simulink model "setPID"  (R2016a)
settings: Solver=FixedStepDiscrete  StartTime=0.0  StopTime=inf  FixedStep=0.005  RelTol=1e-3
PreLoadFcn:
  | if ~exist('Ts', 'var')
  | Ts = 0.001;
  | end
  | if ~exist('Tpwm', 'var')
  | Tpwm = 0.005;
  | end
  | if ~exist('FPGA_Frequency', 'var')
  | FPGA_Frequency = 75000000;
  | end
undefined symbols (not defined in the file or in its folder): IO3xx
libraries: speedgoatlib_fpga x6, slrtlib x3, simulink x1
settings Model: Creator=cedric  LastModifiedBy=kqp5516
settings SolverCC: EnableConcurrentExecution=on
settings DataIOCC: SaveFormat=StructureWithTime
settings OptimizationCC: BlockReduction=off  OptimizeBlockIOStorage=off  BufferReuse=off  GlobalBufferReuse=off  ExpressionFolding=off  LocalBlockOutputs=off
settings DebuggingCC: UnderspecifiedInitializationDetection=Classic  MergeDetectMultiDrivingBlocksExec=none  UnconnectedInputMsg=none  UnconnectedOutputMsg=none  UnconnectedLineMsg=none  SFUnexpectedBacktrackingDiag=error  SFNoUnconditionalDefaultTransitionDiag=error
settings HardwareCC: ProdBitPerPointer=32  ProdLargestAtomicFloat=None  ProdWordSize=32  ProdHWDeviceType=Generic->32-bit x86 compatible
settings ModelReferenceCC: PropagateSignalLabelsOutOfModel=off
settings RTWCC: SystemTargetFile=slrt.tlc  TemplateMakefile=slrt_default_tmf  Description=Simulink Real-Time
settings SimulinkRealTimeCC: RL32LogTETModifier=off  xPCisModelTimeout=off  xPCModelTimeoutSecs=20
settings ConfigComp: CovMetricSettings=dwe  CovHtmlReporting=off  CovSaveCumulativeToWorkspaceVar=off  CovSaveSingleToWorkspaceVar=off  CovExternalEMLEnable=on

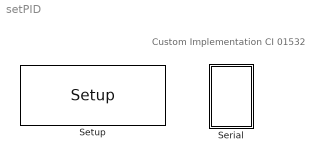
== system setPID ==
  note: Custom Implementation CI 01532
  Serial : Subsystem
  Setup : speedgoatlib_fpga/Setup/Setup  board=IO323  id=1  frontIO=None  rearIO=IO3xx-22  bitstreamFile=speedgoat_IO323_22_CI_01532  ProgSpiFlash=off  ProgBPIFlash=off  pciSlot=-1  PullRPort0=pull-up 3.3V  VioPort0=3.3V  PullRPort1=pull-up 3.3V  VioPort1=3.3V  PullRPort2=pull-up 3.3V  VioPort2=3.3V  PullRPort3=pull-up 3.3V  VioPort3=3.3V  PullRPort4=pull-up 3.3V  VioPort4=3.3V  PullRPort5=pull-up 3.3V  VioPort5=3.3V  PullRPort6=pull-up 3.3V  VioPort6=3.3V  PullRPort15=pull-up 3.3V  PullRPort31=pull-up 3.3V  PullRPort47=pull-up 3.3V  PullRPort63=pull-up 3.3V

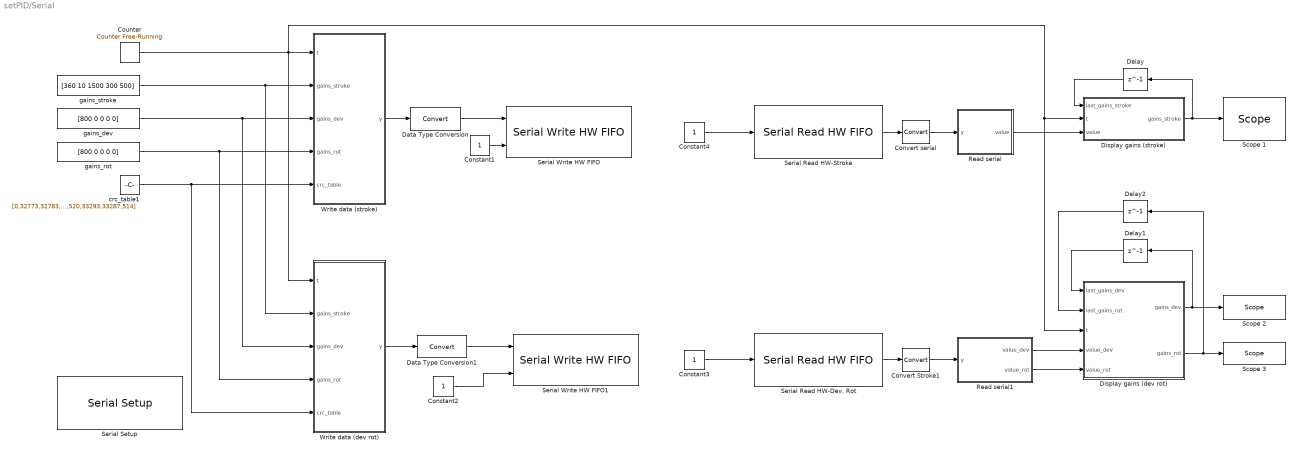
== system setPID/Serial ==
  Constant{1..4} (4 alike) : Constant  OutDataTypeStr=Inherit: Inherit via back propagation
  Convert Stroke1 : DataTypeConversion
  Convert serial : DataTypeConversion
  Counter : simulink/Sources/Counter Free-Running  NumBits=16  tsamp=-1
  Data Type Conversion : DataTypeConversion
  Data Type Conversion1 : DataTypeConversion
  Delay : Delay  DelayLength=1  InitialCondition=zeros(1,5)
  Delay1 : Delay  DelayLength=1  InitialCondition=zeros(1,5)
  Delay2 : Delay  DelayLength=1  InitialCondition=zeros(1,5)
  Display gains (dev rot) : MATLAB Function  TreatAsAtomicUnit=on
  Display gains (stroke) : MATLAB Function  TreatAsAtomicUnit=on
  Read serial : MATLAB Function  TreatAsAtomicUnit=on
  Read serial1 : MATLAB Function  TreatAsAtomicUnit=on
  Scope 1 : slrtlib/Displays and Logging/Scope   scopeno=1  scopetype=Target  autostart=on  viewmode=Numerical  formatstr='%15.0f,%15.0f,%15.0f,%15.0f,%15.0f'  grid=on  ylimits=[0,0]  nosamples=100  noprepostsamples=0  interleave=1  triggermode=FreeRun  triggersignal=1  trigsignalfromport=off  triggerlevel=0.0  triggerslope=Either  triggerscope=1  triggersample=0  filename=data.dat  mode=Lazy  writesize=512  autorestart=off  dynamicfilemode=off  maxwritefilesize=512*1024^2
  Scope 2 : slrtlib/Displays and Logging/Scope   scopeno=2  scopetype=Target  autostart=on  viewmode=Numerical  formatstr='%15.0f,%15.0f,%15.0f,%15.0f,%15.0f'  grid=on  ylimits=[0,0]  nosamples=100  noprepostsamples=0  interleave=1  triggermode=FreeRun  triggersignal=1  trigsignalfromport=off  triggerlevel=0.0  triggerslope=Either  triggerscope=1  triggersample=0  filename=data.dat  mode=Lazy  writesize=512  autorestart=off  dynamicfilemode=off  maxwritefilesize=512*1024^2
  Scope 3 : slrtlib/Displays and Logging/Scope   scopeno=3  scopetype=Target  autostart=on  viewmode=Numerical  formatstr='%15.0f,%15.0f,%15.0f,%15.0f,%15.0f'  grid=on  ylimits=[0,0]  nosamples=100  noprepostsamples=0  interleave=1  triggermode=FreeRun  triggersignal=1  trigsignalfromport=off  triggerlevel=0.0  triggerslope=Either  triggerscope=1  triggersample=0  filename=data.dat  mode=Lazy  writesize=512  autorestart=off  dynamicfilemode=off  maxwritefilesize=512*1024^2
  Serial Read HW-Dev. Rot : speedgoatlib_fpga/Serial/Serial Read HW FIFO  id=1  channel=6  board=IO323  nb_data_bits=8  pciSlot=-1  ts=0.005
  Serial Read HW-Stroke : speedgoatlib_fpga/Serial/Serial Read HW FIFO  id=1  channel=1  board=IO323  nb_data_bits=8  pciSlot=-1  ts=0.005
  Serial Setup : speedgoatlib_fpga/Serial/Serial Setup  id=1  channel=[1 6]  bitrate_configuration=Simple  bitrate=[1000000]  bitrate_effective=[1e6, 1e6]  bitrate_error=[0, 0]  base_clock=[75000000, 75000000]  divider=[5, 5]  cpr=[1, 1]  tcr=[15, 15]  parity=No parity  nb_data_bits=[8]  nb_stop_bits=[1]  rs485_half_duplex=on  board=IO323  pciSlot=-1
  Serial Write HW FIFO : speedgoatlib_fpga/Serial/Serial Write HW FIFO  id=1  channel=1  board=IO323  tx_fifo_mode=Halt model on buffer overflow  nb_data_bits=8  pciSlot=-1  ts=0.005
  Serial Write HW FIFO1 : speedgoatlib_fpga/Serial/Serial Write HW FIFO  id=1  channel=6  board=IO323  tx_fifo_mode=Halt model on buffer overflow  nb_data_bits=8  pciSlot=-1  ts=0.005
  Write data (dev rot) : MATLAB Function  TreatAsAtomicUnit=on
  Write data (stroke) : MATLAB Function  TreatAsAtomicUnit=on
  crc_table1 : Constant  Value=[0,32773,32783,10,32795,30,20,32785,32819,54,60,32825,40,32813,32807,34,32867,102,108,32873,120,32893,32887,114,80,32853,32863,90,32843,78,68,32833,32963,198,204,32969,216,32989,32983,210,240,33013,33023,250,33003,238,228,32993,160,32933,32943,170,32955,190,180,32945,32915,150,156,32921,136,32909,32903,130,33155,390,396,33161,408,33181,33175,402,432,33205,33215,442,33195,430,420,33185,480,33253,33263,490,33275,510,500,33265,33235,470,476,33241,456,33229,33223,450,320,33093,33103,330,33115,350,340,33105,33139,374,380,33145,360,33133,33127,354,33059,294,300,33065,312,33085,33079,306,272,33045,33055,282,33035,270,260,33025,33539,774,780,33545,792,33565,33559,786,816,33589,33599,826,33579,814,804,33569,864,33637,33647,874,33659,894,884,33649,33619,854,860,33625,840,33613,33607,834,960,33733,33743,970,33755,990,980,33745,33779,1014,1020,33785,1000,33773,33767,994,33699,934,940,33705,952,33725,33719,946,912,33685,33695,922,33675,910,900,33665,640,33413,33423,650,33435,670,660,33425,33459,694,700,33465,680,33453,33447,674,33507,742,748,33513,760,33533,33527,754,720,33493,33503,730,33483,718,708,33473,33347,582,588,33353,600,33373,33367,594,624,33397,33407,634,33387,622,612,33377,544,33317,33327,554,33339,574,564,33329,33299,534,540,33305,520,33293,33287,514]  OutDataTypeStr=Inherit: Inherit via back propagation
  gains_dev : Constant  Value=[800 0 0 0 0]
  gains_rot : Constant  Value=[800 0 0 0 0]
  gains_stroke : Constant  Value=[360 10 1500 300 500]
  wires:
  Constant1/1 -> Serial Write HW FIFO/2
  Data Type Conversion/1 -> Serial Write HW FIFO/1
  Write data (stroke)/1(y) -> Data Type Conversion/1
  Constant2/1 -> Serial Write HW FIFO1/2
  Data Type Conversion1/1 -> Serial Write HW FIFO1/1
  crc_table1/1 -> Write data (dev rot)/5(crc_table), Write data (stroke)/5(crc_table)
  Constant3/1 -> Serial Read HW-Dev. Rot/1
  Constant4/1 -> Serial Read HW-Stroke/1
  Serial Read HW-Stroke/1 -> Convert serial/1
  Serial Read HW-Dev. Rot/1 -> Convert Stroke1/1
  Convert serial/1 -> Read serial/1(y)
  Convert Stroke1/1 -> Read serial1/1(y)
  gains_stroke/1 -> Write data (dev rot)/2(gains_stroke), Write data (stroke)/2(gains_stroke)
  Counter/1 -> Write data (dev rot)/1(t), Write data (stroke)/1(t), Display gains (stroke)/2(t), Display gains (dev rot)/3(t)
  gains_dev/1 -> Write data (dev rot)/3(gains_dev), Write data (stroke)/3(gains_dev)
  gains_rot/1 -> Write data (dev rot)/4(gains_rot), Write data (stroke)/4(gains_rot)
  Delay/1 -> Display gains (stroke)/1(last_gains_stroke)
  Display gains (stroke)/1(gains_stroke) -> Scope 1/1, Delay/1
  Read serial/1(value) -> Display gains (stroke)/3(value)
  Write data (dev rot)/1(y) -> Data Type Conversion1/1
  Delay1/1 -> Display gains (dev rot)/1(last_gains_dev)
  Display gains (dev rot)/1(gains_dev) -> Delay1/1, Scope 2/1
  Read serial1/1(value_dev) -> Display gains (dev rot)/4(value_dev)
  Display gains (dev rot)/2(gains_rot) -> Scope 3/1, Delay2/1
  Delay2/1 -> Display gains (dev rot)/2(last_gains_rot)
  Read serial1/2(value_rot) -> Display gains (dev rot)/5(value_rot)

== matlab function setPID/Serial/Write data (stroke) ==
  data: y output; t input; gains_stroke input; gains_dev input; gains_rot input; crc_table input
function y = fcn(t,gains_stroke,gains_dev,gains_rot,crc_table)
%#codegen
y = zeros(1,129);
% y = packetMultiWritePID(30,1,0,crc_table);
%% READ
if mod(t,10) == 0 % read P gain
    y = packetMultiWritePID(30,1,0,crc_table);
elseif mod(t,10) == 1 % read I gain
    y = packetMultiWritePID(40,1,0,crc_table);
elseif mod(t,10) == 2 % read D gain
    y = packetMultiWritePID(50,1,0,crc_table);
elseif mod(t,10) == 3 % read Profile Acceleration
    y = packetMultiWritePID(60,1,0,crc_table);
elseif mod(t,10) == 4 % read Profile Velocity
    y = packetMultiWritePID(70,1,0,crc_table);
%% WRITE
elseif mod(t,10) == 5 % write P gain
    y = packetMultiWritePID(32,[1 2 3],[gains_stroke(1),gains_dev(1),gains_rot(1)],crc_table);
elseif mod(t,10) == 6 % write I gain
    y = packetMultiWritePID(42,[1 2 3],[gains_stroke(2),gains_dev(2),gains_rot(2)],crc_table);
elseif mod(t,10) == 7 % write D gain
    y = packetMultiWritePID(52,[1 2 3],[gains_stroke(3),gains_dev(3),gains_rot(3)],crc_table);
elseif mod(t,10) == 8 % write Profile Acceleration
    y = packetMultiWritePID(62,[1 2 3],[gains_stroke(4),gains_dev(4),gains_rot(4)],crc_table);
elseif mod(t,10) == 9 % write Profile Velocity
    y = packetMultiWritePID(72,[1 2 3],[gains_stroke(5),gains_dev(5),gains_rot(5)],crc_table);
end

end

== matlab function setPID/Serial/Display gains (stroke) ==
  data: last_gains_stroke input; t input; value input; gains_stroke output
function gains_stroke = fcn(last_gains_stroke,t,value)
%#codegen
gains_stroke = last_gains_stroke;
%% READ
if mod(t,10) == 1 % read P gain
    gains_stroke(1) = value;
elseif mod(t,10) == 2 % read I gain
    gains_stroke(2) = value;
elseif mod(t,10) == 3 % read D gain
    gains_stroke(3) = value;
elseif mod(t,10) == 4 % read Profile Acceleration
    gains_stroke(4) = value;
elseif mod(t,10) == 5 % read Profile Velocity
    gains_stroke(5) = value;
end
end

== matlab function setPID/Serial/Write data (dev rot) ==
  data: y output; t input; gains_stroke input; gains_dev input; gains_rot input; crc_table input
function y = fcn(t,gains_stroke,gains_dev,gains_rot,crc_table)
%#codegen
y = zeros(1,129);
% y = packetMultiWritePID(30,1,0,crc_table);
%% READ
if mod(t,10) == 0 % read P gain
    y = packetMultiWritePID(31,[1 2 3],0,crc_table);
elseif mod(t,10) == 1 % read I gain
    y = packetMultiWritePID(41,[1 2 3],0,crc_table);
elseif mod(t,10) == 2 % read D gain
    y = packetMultiWritePID(51,[1 2 3],0,crc_table);
elseif mod(t,10) == 3 % read Profile Acceleration
    y = packetMultiWritePID(61,[1 2 3],0,crc_table);
elseif mod(t,10) == 4 % read Profile Velocity
    y = packetMultiWritePID(71,[1 2 3],0,crc_table);
%% WRITE
elseif mod(t,10) == 5 % write P gain
    y = packetMultiWritePID(32,[1 2 3],[gains_stroke(1),gains_dev(1),gains_rot(1)],crc_table);
elseif mod(t,10) == 6 % write I gain
    y = packetMultiWritePID(42,[1 2 3],[gains_stroke(2),gains_dev(2),gains_rot(2)],crc_table);
elseif mod(t,10) == 7 % write D gain
    y = packetMultiWritePID(52,[1 2 3],[gains_stroke(3),gains_dev(3),gains_rot(3)],crc_table);
elseif mod(t,10) == 8 % write Profile Acceleration
    y = packetMultiWritePID(62,[1 2 3],[gains_stroke(4),gains_dev(4),gains_rot(4)],crc_table);
elseif mod(t,10) == 9 % write Profile Velocity
    y = packetMultiWritePID(72,[1 2 3],[gains_stroke(5),gains_dev(5),gains_rot(5)],crc_table);
end

end

== matlab function setPID/Serial/Display gains (dev rot) ==
  data: last_gains_dev input; last_gains_rot input; t input; value_dev input; gains_dev output; gains_rot output; value_rot input
function [gains_dev,gains_rot] = fcn(last_gains_dev,last_gains_rot,t,value_dev,value_rot)
%#codegen
gains_dev = last_gains_dev;
gains_rot = last_gains_rot;
%% READ
if mod(t,10) == 1 % read P gain
    gains_dev(1) = value_dev;
    gains_rot(1) = value_rot;
elseif mod(t,10) == 2 % read I gain
    gains_dev(2) = value_dev;
    gains_rot(2) = value_rot;
elseif mod(t,10) == 3 % read D gain
    gains_dev(3) = value_dev;
    gains_rot(3) = value_rot;
elseif mod(t,10) == 4 % read Profile Acceleration
    gains_dev(4) = value_dev;
    gains_rot(4) = value_rot;
elseif mod(t,10) == 5 % read Profile Velocity
    gains_dev(5) = value_dev;
    gains_rot(5) = value_rot;
end
end

== matlab function setPID/Serial/Read serial1 ==
  data: y input; value_dev output; value_rot output
function [value_dev,value_rot] = fcn(y)
%#codegen
value_dev = 0;
value_rot = 0;
ID = [1 2 3];
for i = 1:1:length(y)-5
    % dev
    if y(i) == 255 && y(i+1) == 255 && y(i+2) == 253 && y(i+4) == ID(2) && y(i+5) == 6 % packet length 6 b/c: 2 params (bytes) + 1 error byte + 3
        temp = i;
        Para = y(temp+9:temp+10); % 2 params only
        value_dev = byte_to_num16(Para);    
    elseif y(i) == 255 && y(i+1) == 255 && y(i+2) == 253 && y(i+4) == ID(2) && y(i+5) == 8 % packet length 8 b/c: 4 params (bytes) + 1 error byte + 3
        temp = i;
        Para = y(temp+9:temp+12); % 4 params
        value_dev = byte_to_num32(Para);
    % rot
    elseif y(i) == 255 && y(i+1) == 255 && y(i+2) == 253 && y(i+4) == ID(3) && y(i+5) == 6 % packet length 6 b/c: 2 params (bytes) + 1 error byte + 3
        temp = i;
        Para = y(temp+9:temp+10); % 2 params only
        value_rot = byte_to_num16(Para);    
    elseif y(i) == 255 && y(i+1) == 255 && y(i+2) == 253 && y(i+4) == ID(3) && y(i+5) == 8 % packet length 8 b/c: 4 params (bytes) + 1 error byte + 3
        temp = i;
        Para = y(temp+9:temp+12); % 4 params
        value_rot = byte_to_num32(Para);
    end
end

end

function value_byte = byte_to_num16(para)
value_byte = double(typecast(uint8(para),'uint16')); % uint16 instead of uint32
end

function value_byte = byte_to_num32(para)
value_byte = double(typecast(uint8(para),'uint32'));
end

== matlab function setPID/Serial/Read serial ==
  data: y input; value output
function value = fcn(y)
%#codegen
value = 0;
ID = 1;
for i = 1:1:length(y)-5
    if y(i) == 255 && y(i+1) == 255 && y(i+2) == 253 && y(i+4) == ID && y(i+5) == 6 % packet length 6 b/c: 2 params (bytes) + 1 error byte + 3
        temp = i;
        Para = y(temp+9:temp+10); % 2 params only
        value = byte_to_num16(Para);    
    elseif y(i) == 255 && y(i+1) == 255 && y(i+2) == 253 && y(i+4) == ID && y(i+5) == 8 % packet length 8 b/c: 4 params (bytes) + 1 error byte + 3
        temp = i;
        Para = y(temp+9:temp+12); % 4 params
        value = byte_to_num32(Para);
    end
end

end

function value_byte = byte_to_num16(para)
value_byte = double(typecast(uint8(para),'uint16')); % uint16 instead of uint32
end

function value_byte = byte_to_num32(para)
value_byte = double(typecast(uint8(para),'uint32'));
end
